simulink model "RTW_2_round_system"  (R2016a)
settings: Solver=ode5  StartTime=0.0  StopTime=10  FixedStep=0.001  RelTol=1e-3
values from neighbouring files (symbols this model uses):
  LK1 = [-1 0;0 -1]    [RTW_2_round_system_m.m]    (also in RTW_3_cluster_follow_system_m.m = -LK1; car_m.m = [-1 0;0 -1]')
  x0 = [0 0]'    [RTW_2_round_system_m.m]    (also in RTW_3_cluster_follow_system_m.m = x0'; car_m.m = [1 3]')
  xd = [10 10]    [RTW_2_round_system_m.m]    (also in RTW_3_cluster_follow_system_m.m = [0 0 0 0 0 0 0 0]; car_m.m)
libraries: simulink x1
settings Model: Creator=108  LastModifiedBy=richa

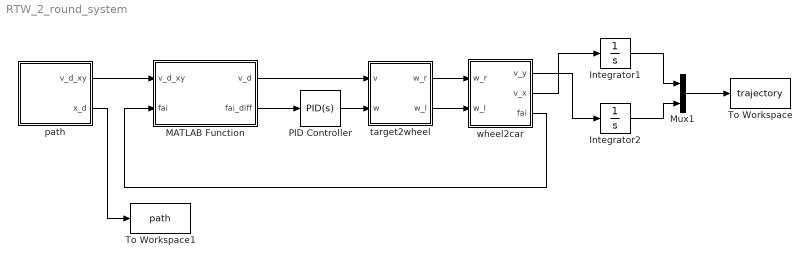
== system RTW_2_round_system ==
  Integrator1 : Integrator
  Integrator2 : Integrator
  MATLAB Function : MATLAB Function  TreatAsAtomicUnit=on
  Mux1 : Mux  Inputs=2
  PID Controller : simulink/Continuous/PID Controller  Controller=PID  TimeDomain=Continuous-time  SampleTime=-1  IntegratorMethod=Forward Euler  FilterMethod=Forward Euler  Form=Parallel  UseFilter=on  ControllerParametersSource=internal  P=200  I=10  D=0  N=100  InitialConditionSource=internal  InitialConditionForIntegrator=0  InitialConditionForFilter=0  ExternalReset=none  LimitOutput=off  UpperSaturationLimit=inf  LowerSaturationLimit=-inf  LinearizeAsGain=on  AntiWindupMode=none  Kb=1  TrackingMode=off  Kt=1  PParamMin=[]  PParamMax=[]  IParamMin=[]  IParamMax=[]  DParamMin=[]  DParamMax=[]  NParamMin=[]  NParamMax=[]  KbParamMin=[]  KbParamMax=[]  KtParamMin=[]  KtParamMax=[]  POutMin=[]  POutMax=[]  IOutMin=[]  IOutMax=[]  DOutMin=[]  DOutMax=[]  NOutMin=[]  NOutMax=[]  KbOutMin=[]  KbOutMax=[]  KtOutMin=[]  KtOutMax=[]  IntegratorOutMin=[]  IntegratorOutMax=[]  FilterOutMin=[]  FilterOutMax=[]  SumOutMin=[]  SumOutMax=[]  SumI1OutMin=[]  SumI1OutMax=[]  SumI2OutMin=[]  SumI2OutMax=[]  SumI3OutMin=[]  SumI3OutMax=[]  SumDOutMin=[]  SumDOutMax=[]  SaturationOutMin=[]  SaturationOutMax=[]  IntegratorContinuousStateAttributes=''  IntegratorStateMustResolveToSignalObject=off  IntegratorRTWStateStorageClass=Auto  FilterContinuousStateAttributes=''  FilterStateMustResolveToSignalObject=off  FilterRTWStateStorageClass=Auto  DifferentiatorICPrevScaledInput=0  DifferentiatorOutMin=[]  DifferentiatorOutMax=[]
  To Workspace : ToWorkspace  VariableName=trajectory  SampleTime=-1
  To Workspace1 : ToWorkspace  VariableName=path  SampleTime=-1
  path : Subsystem
  target2wheel : Subsystem
  wheel2car : Subsystem
  wires:
  Integrator1/1 -> Mux1/1
  Integrator2/1 -> Mux1/2
  target2wheel/1(w_r) -> wheel2car/1(w_r)
  target2wheel/2(w_l) -> wheel2car/2(w_l)
  MATLAB Function/2(fai_diff) -> PID Controller/1
  PID Controller/1 -> target2wheel/2(w)
  wheel2car/3(fai) -> MATLAB Function/2(fai)
  Mux1/1 -> To Workspace/1
  wheel2car/2(v_x) -> Integrator1/1
  wheel2car/1(v_y) -> Integrator2/1
  MATLAB Function/1(v_d) -> target2wheel/1(v)
  path/2(x_d) -> To Workspace1/1
  path/1(v_d_xy) -> MATLAB Function/1(v_d_xy)

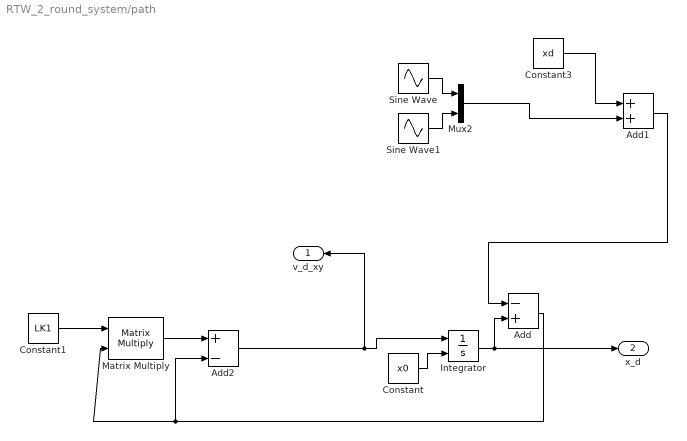
== system RTW_2_round_system/path ==
  Add : Sum  Inputs=-+
  Add1 : Sum
  Add2 : Sum  Inputs=+-
  Constant : Constant  Value=x0
  Constant1 : Constant  Value=LK1  VectorParams1D=off
  Constant3 : Constant  Value=xd
  Integrator : Integrator  InitialConditionSource=external
  Matrix Multiply : Product  Multiplication=Matrix(*)
  Mux2 : Mux  Inputs=2
  Sine Wave : Sin  Amplitude=10  SampleTime=0
  Sine Wave1 : Sin  Amplitude=10  Phase=pi/2  SampleTime=0
  v_d_xy : Outport
  x_d : Outport  Port=2
  wires:
  Matrix Multiply/1 -> Add2/1
  Integrator/1 -> x_d/1, Add/2
  Constant/1 -> Integrator/2
  Constant1/1 -> Matrix Multiply/1
  Add/1 -> Add2/2, Matrix Multiply/2
  Add2/1 -> Integrator/1, v_d_xy/1
  Sine Wave/1 -> Mux2/1
  Sine Wave1/1 -> Mux2/2
  Constant3/1 -> Add1/1
  Mux2/1 -> Add1/2
  Add1/1 -> Add/1

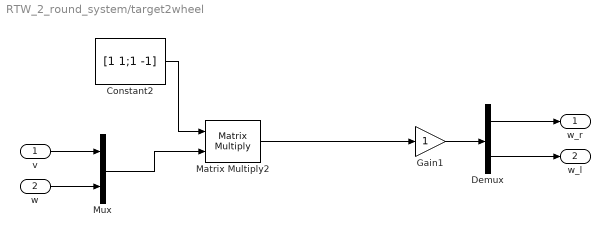
== system RTW_2_round_system/target2wheel ==
  v : Inport
  w : Inport  Port=2
  Constant2 : Constant  Value=[1 1;1 -1]
  Demux : Demux  Outputs=2
  Gain1 : Gain
  Matrix Multiply2 : Product  Multiplication=Matrix(*)
  Mux : Mux  Inputs=2
  w_r : Outport
  w_l : Outport  Port=2
  wires:
  Mux/1 -> Matrix Multiply2/2
  Gain1/1 -> Demux/1
  Constant2/1 -> Matrix Multiply2/1
  Matrix Multiply2/1 -> Gain1/1
  v/1 -> Mux/1
  w/1 -> Mux/2
  Demux/2 -> w_l/1
  Demux/1 -> w_r/1

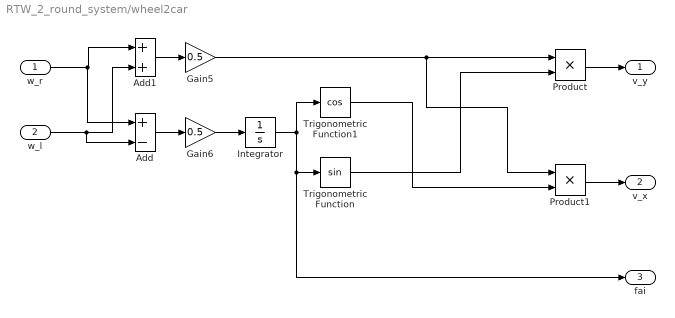
== system RTW_2_round_system/wheel2car ==
  w_r : Inport
  w_l : Inport  Port=2
  Add : Sum  Inputs=+-
  Add1 : Sum
  Gain5 : Gain  Gain=0.5
  Gain6 : Gain  Gain=0.5
  Integrator : Integrator
  Product : Product
  Product1 : Product
  Trigonometric Function : Trigonometry
  Trigonometric Function1 : Trigonometry  Operator=cos
  v_y : Outport
  v_x : Outport  Port=2
  fai : Outport  Port=3
  wires:
  Gain5/1 -> Product1/1, Product/1
  Gain6/1 -> Integrator/1
  Integrator/1 -> Trigonometric Function1/1, fai/1, Trigonometric Function/1
  Trigonometric Function/1 -> Product/2
  Trigonometric Function1/1 -> Product1/2
  w_r/1 -> Add/1, Add1/1
  w_l/1 -> Add/2, Add1/2
  Add1/1 -> Gain5/1
  Add/1 -> Gain6/1
  Product1/1 -> v_x/1
  Product/1 -> v_y/1

== matlab function RTW_2_round_system/MATLAB Function ==
  data: v_d_xy input; v_d output; fai_diff output; fai input
function [v_d,fai_diff]  = fcn(v_d_xy,fai)
%#codegen

v_d=[0];
fai_diff=[0];
j=1;

for i=1:1
    v_d(j) = sqrt(v_d_xy(i).^2+ v_d_xy(i+1).^2);
    fai_d = atan2(v_d_xy(i+1),v_d_xy(i));
    fai_diff(j)= fai_d-fai;
    if fai_diff(j)>pi
        fai_diff(j)=fai_diff(j)-2*pi*round(fai_diff(j)/(2*pi));
    elseif fai_diff(j)<-pi
        fai_diff(j)=fai_diff(j)+2*pi*round(fai_diff(j)/(-2*pi));      
    end
   
   j=j+1;
end

end
